simulink subsystem "MCuC"  (R2023b)
settings: Solver=VariableStepAuto  StartTime=0.0  StopTime=10.0  RelTol=1e-3
settings Model: Creator=nickj  LastModifiedBy=heyka

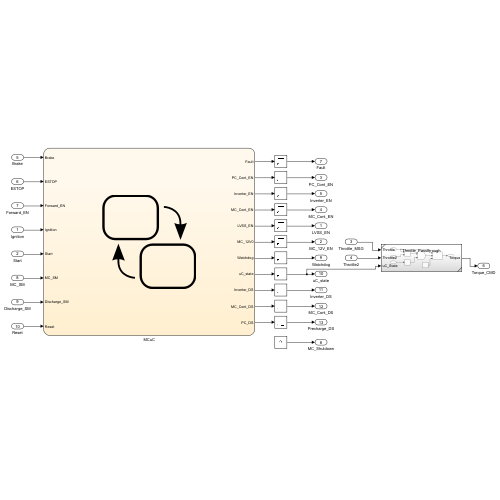
[thumbnail: Simulink's stored preview of the top-level diagram]
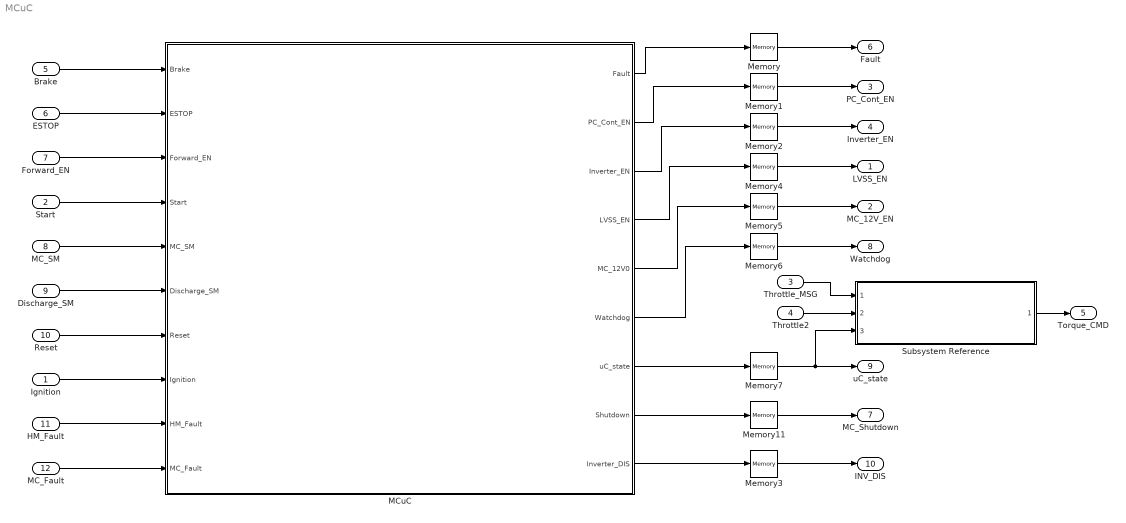
== system MCuC ==
  Ignition : Inport
  Start : Inport  Port=2
  Throttle_MSG : Inport  Port=3
  Throttle2 : Inport  Port=4
  Brake : Inport  Port=5
  ESTOP : Inport  Port=6
  Forward_EN : Inport  Port=7
  MC_SM : Inport  Port=8
  Discharge_SM : Inport  Port=9
  Reset : Inport  Port=10
  HM_Fault : Inport  Port=11
  MC_Fault : Inport  Port=12
  MCuC : Stateflow chart  TreatAsAtomicUnit=on
      settings: PortSchema="{\"entries\":[{\"content\":{\"sides\":[{\"content\":{\"connectorIds\":[\"In1\",\"In2\",\"In3\",\"In5\",\"In6\",\"In7\",\"In8\",\"In4\",\"In9\",\"In10\"]},\"type\":\"ConnectorPlacement.EquallySpacedRectSide\",\"uuid\":\"d1510c73-f1c7-4e03-bb6c-bda7856f993e\"},{\"content\":{\"connectorIds\":[\"Out1\",\"Out2\",\"Out3\",\"Out4\",\"Out5\",\"Out6\",\"Out7\",\"Out8\",\"Out9\"],\"side\":\"RIGHT\"},\"type\":\"ConnectorPlacement.EquallySpacedRectSide\",\"uuid\":\"1a7878c4-a817-4ca0-b21c-0429e82bb9d7\"},{\"content\":{\"side\":\"TOP\"},\"type\":\"ConnectorPlacement.EquallySpacedRectSide\",\"uuid\":\"ed9f2701-7044-4bb4-9c0b-b9cf9840e69e\"}]},\"type\":\"ConnectorPlacement.EquallySpacedConnector\",\"uuid\":\"4ceb8e7d-629c-4438-88a9-aa3016537644\"}],\"packageUris\":[\"http://schema.mathworks.com/mf0/Connector/R2020b\"],\"version\":\"1.0\"}"
  Memory{,1..7,11} (9 alike) : Memory
  Subsystem Reference : Subsystem  ReferencedSubsystem=Throttle_Passthrough
  LVSS_EN : Outport
  MC_12V_EN : Outport  Port=2
  PC_Cont_EN : Outport  Port=3
  Inverter_EN : Outport  Port=4
  Torque_CMD : Outport  Port=5
  Fault : Outport  Port=6
  MC_Shutdown : Outport  Port=7
  Watchdog : Outport  Port=8
  uC_state : Outport  Port=9
  INV_DIS : Outport  Port=10
  wires:
  Memory7/1 -> Subsystem Reference/3, uC_state/1
  Brake/1 -> MCuC/1(Brake)
  Discharge_SM/1 -> MCuC/7(Discharge_SM)
  ESTOP/1 -> MCuC/2(ESTOP)
  Forward_EN/1 -> MCuC/3(Forward_EN)
  MCuC/8(Shutdown) -> Memory11/1
  Start/1 -> MCuC/5(Start)
  Reset/1 -> MCuC/8(Reset)
  MC_SM/1 -> MCuC/6(MC_SM)
  Ignition/1 -> MCuC/4(Ignition)
  Memory4/1 -> LVSS_EN/1
  HM_Fault/1 -> MCuC/9(HM_Fault)
  Memory6/1 -> Watchdog/1
  MC_Fault/1 -> MCuC/10(MC_Fault)
  MCuC/1(Fault) -> Memory/1
  MCuC/2(PC_Cont_EN) -> Memory1/1
  MCuC/3(Inverter_EN) -> Memory2/1
  Memory2/1 -> Inverter_EN/1
  MCuC/4(LVSS_EN) -> Memory4/1
  MCuC/5(MC_12V0) -> Memory5/1
  MCuC/6(Watchdog) -> Memory6/1
  MCuC/7(uC_state) -> Memory7/1
  MCuC/9(Inverter_DIS) -> Memory3/1
  Memory/1 -> Fault/1
  Memory1/1 -> PC_Cont_EN/1
  Memory5/1 -> MC_12V_EN/1
  Throttle_MSG/1 -> Subsystem Reference/1
  Throttle2/1 -> Subsystem Reference/2
  Memory11/1 -> MC_Shutdown/1
  Memory3/1 -> INV_DIS/1
  Subsystem Reference/1 -> Torque_CMD/1

== stateflow chart MCuC/MCuC ==
  state MCuC
    state MCuC_Logic [parallel]
      settings: executionOrder=1
      state ESTOP
        entry:
        uC_state = 7;
        MC_12V0 = 0;
        ESTOP_activated = 0;
      state MC_Off
        entry:
        MC_12V0 = 0;
        uC_state = 0;
        uncharged = 1;
      state MC_Discharging
        entry:
        uC_state = 5;
        state LVSS_EN_OFF
          entry:
          LVSS_EN = 0
        state LVSS_EN_ON
          entry:
          LVSS_EN = 1;
        (default) -> LVSS_EN_ON
        LVSS_EN_ON -> LVSS_EN_OFF : after(Pulse, sec)
        MC_Discharging -> LVSS_EN_ON : [Discharge_SM ==4]
      state Fault
        entry:
        uC_state = 6;
        state LVSS_DIS_OFF
          LVSS_EN = 0;
        state Fault_OFF
          Fault = 0;
        state LVSS_DIS_ON
          LVSS_EN = 1;
        state Fault_ON
          Fault =1;
        LVSS_DIS_ON -> LVSS_DIS_OFF : after(Pulse, sec)
        Fault_OFF -> LVSS_DIS_ON [order 2] : [Ignition == 0]
        Fault_ON -> Fault_OFF : after(Pulse, sec)
        (default) -> Fault_ON
      state MC_Init
        entry:
        uncharged = 0;
        uC_state = 1;
        MC_12V0 = 1;
        state POWER_EN_ON
          LVSS_EN = 1;
          PC_Cont_EN =1;
        state POWER_EN_OFF
          LVSS_EN = 0;
          PC_Cont_EN = 0;
        (default) -> POWER_EN_ON
        POWER_EN_ON -> POWER_EN_OFF : after(Pulse, sec)
        POWER_EN_OFF -> (junction 271)
      state Contactor_Open
        entry:
        Inverter_DIS = 0
        uC_state = 4;
        state Shutdown_On
          Shutdown = 1
        state Shutdown_Off
          Shutdown = 0
        (default) -> Shutdown_On
        Shutdown_On -> Shutdown_Off : after(Pulse, sec)
      state MC_Active
        entry:
        uC_state = 3;
        state INV_DS_OFF
          Inverter_DIS = 0;
        state INV_DIS_ON
          Inverter_DIS = 1;
        state INV_EN_ON
          Inverter_EN = 1;
        state INV_EN_OFF
          Inverter_EN = 0;
        INV_DS_OFF -> (junction 240)
        INV_DIS_ON -> INV_DS_OFF : after(Pulse, sec)
        INV_EN_OFF -> INV_DIS_ON : [Forward_EN == 0 || Ignition == 0]
        (default) -> INV_EN_ON
        INV_EN_ON -> INV_EN_OFF : after(Pulse, sec)
      state Contactor_Closed
        entry:
        uC_state = 2;
      MCuC_Logic -> MC_Off [order 5] : [Reset == 1]
      (default) -> MC_Off
      ESTOP -> MC_Off : [ESTOP == 0]
      MCuC_Logic -> ESTOP [order 3] : [ESTOP == 1 && uncharged == 1]
      Fault_OFF -> MC_Off [order 1] : [MC_12V0 == 0 && Ignition == 0]
      LVSS_EN_OFF -> MC_Off
      LVSS_DIS_OFF -> MC_Off
      MC_Off -> MC_Init : [Ignition == 1]
      Shutdown_Off -> MC_Discharging : [Discharge_SM == 3]
      MCuC_Logic -> Fault [order 4] : [HM_Fault == 1 && Ignition == 1]
      MCuC_Logic -> Fault [order 2] : [MC_Fault == 1 && Ignition == 1]
      MCuC_Logic -> Contactor_Open [order 1] : [ESTOP == 1 && uncharged == 0 && ESTOP_activated == 0]{ESTOP_activated = 1}
      (junction 271) -> Contactor_Open [order 1] : [Ignition == 0]
      (junction 271) -> Contactor_Closed [order 2] : [MC_SM == 4]
      Contactor_Closed -> Contactor_Open [order 2] : [Ignition == 0]
      (junction 240) -> Contactor_Open [order 1] : [Ignition == 0]
      Contactor_Closed -> MC_Active [order 1] : [Start == 1 && Forward_EN == 1 && Brake == 1]
      (junction 240) -> Contactor_Closed [order 2] : [Forward_EN == 0]
    state Watchdog [parallel]
      settings: executionOrder=2
      state WD0
        entry:
        Watchdog = 0;
      state WD1
        entry:
        Watchdog = 1;
      (default) -> WD0
      WD0 -> WD1 : after(.5, sec)
      WD1 -> WD0
  data: Fault output =0; PC_Cont_EN output =0; Brake input; ESTOP input; Forward_EN input; Ignition input; Start input; MC_SM input; Inverter_EN output =0; LVSS_EN output =0; MC_12V0 output =0; Discharge_SM input; Reset input; Watchdog output =0; uC_state output; Pulse local =0.01; Shutdown output; uncharged local; Inverter_DIS output; ESTOP_activated local =0; HM_Fault input; MC_Fault input
